simulink model "inputSignals"  (R2019a)
settings: Solver=VariableStepAuto  StartTime=0.0  StopTime=300  RelTol=1e-3
settings Model: Creator=Dario Quintero  LastModifiedBy=dq16394
settings DebuggingCC: ArithmeticOperatorsInVariantConditions=warning

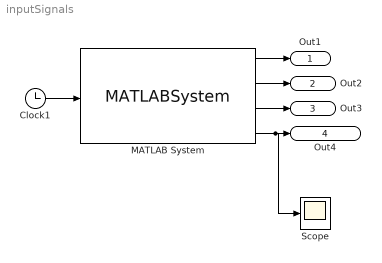
== system inputSignals ==
  Clock1 : Clock
  MATLAB System : MATLABSystem  System=HeadingSignals  SimulateUsing=Interpreted execution
      mask Type: HeadingSignals
      mask Display:
      | disp('HeadingSignals');
      | port_label('input',1,'time');
      | port_label('output',1,'step');
      | port_label('output',2,'ramp');
      | port_label('output',3,'sine');
      | port_label('output',4,'trueHeading');
  Scope : Scope
  Out1 : Outport  SignalName=step
  Out2 : Outport  Port=2  SignalName=ramp
  Out3 : Outport  Port=3  SignalName=sine
  Out4 : Outport  Port=4  SignalName=trueHeading
  wires:
  MATLAB System/1 -> Out1/1
  Clock1/1 -> MATLAB System/1
  MATLAB System/2 -> Out2/1
  MATLAB System/3 -> Out3/1
  MATLAB System/4 -> Out4/1, Scope/1
